simulink model "gm_receive_OK"  (R2015b)
settings: Solver=VariableStepAuto  StartTime=0  StopTime=25  RelTol=1e-3
settings Model: Creator=Administrator  LastModifiedBy=Administrator
settings OptimizationCC: BlockReduction=off  ConditionallyExecuteInputs=off
settings DebuggingCC: InheritedTsInSrcMsg=none

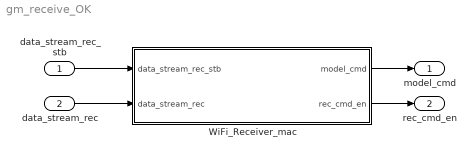
== system gm_receive_OK ==
  data_stream_rec_stb : Inport  OutDataTypeStr=boolean  SampleTime=0
  data_stream_rec : Inport  Port=2  OutDataTypeStr=uint8  SampleTime=0
  WiFi_Receiver_mac : Subsystem
  model_cmd : Outport  OutDataTypeStr=fixdt(0,4,0)
  rec_cmd_en : Outport  Port=2  OutDataTypeStr=boolean
  wires:
  data_stream_rec_stb/1 -> WiFi_Receiver_mac/1(data_stream_rec_stb)
  data_stream_rec/1 -> WiFi_Receiver_mac/2(data_stream_rec)
  WiFi_Receiver_mac/1(model_cmd) -> model_cmd/1
  WiFi_Receiver_mac/2(rec_cmd_en) -> rec_cmd_en/1

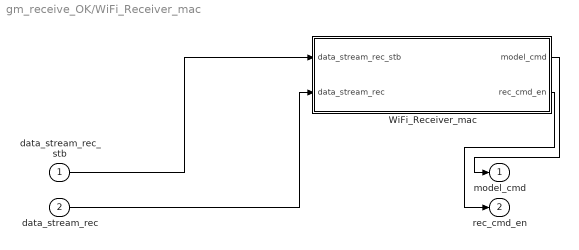
== system gm_receive_OK/WiFi_Receiver_mac ==
  data_stream_rec_stb : Inport  SampleTime=0
  data_stream_rec : Inport  Port=2  SampleTime=0
  WiFi_Receiver_mac : Stateflow chart  TreatAsAtomicUnit=on
  model_cmd : Outport
  rec_cmd_en : Outport  Port=2
  wires:
  data_stream_rec_stb/1 -> WiFi_Receiver_mac/1(data_stream_rec_stb)
  data_stream_rec/1 -> WiFi_Receiver_mac/2(data_stream_rec)
  WiFi_Receiver_mac/1(model_cmd) -> model_cmd/1
  WiFi_Receiver_mac/2(rec_cmd_en) -> rec_cmd_en/1

== stateflow chart gm_receive_OK/WiFi_Receiver_mac/WiFi_Receiver_mac ==
  settings: executeAtInitialization=1
  state wait_cmd
    entry:
    model_cmd=0;
    rec_cmd_en=0;
  state initial
    entry:
    model_cmd=0;
    rec_cmd_en=0;
    time_cnt=0;
  state received_OK
    entry:
    model_cmd=1;
    rec_cmd_en=1;
  state receive_Carriage_Return
  state detect_cmd
  state received_O
  state received_K
  state received_ERROR
    entry:
    model_cmd=2;
    rec_cmd_en=1;
  state time_out
    time_cnt=0;
    model_cmd=2;
    rec_cmd_en=1;
  state received_E
  state received_R
  state received_R1
  state received_O1
  state received_R2
  state receive_Carriage_Return1
  state received_FAIL
    entry:
    model_cmd=3;
    rec_cmd_en=1;
  state received_F
  state received_A
  state received_I
  state received_L
  state receive_Carriage_Return2
  (junction 129) -> wait_cmd
  (junction 152) -> (junction 129)
  (junction 13) -> (junction 129) [order 2] : [data_stream_rec~=75]
  (junction 150) -> (junction 152) [order 2] : [data_stream_rec~=13]
  (junction 22) -> wait_cmd : [(data_stream_rec~=79)&&(data_stream_rec~=69)&&(data_stream_rec~=70)]
  (junction 18) -> (junction 22) [order 2]
  (default) -> initial
  (junction 146) -> received_K [order 2] : [data_stream_rec_stb==0]
  (junction 10) -> received_O [order 1] : [data_stream_rec_stb==0]
  received_OK -> detect_cmd
  receive_Carriage_Return -> received_OK
  (junction 150) -> receive_Carriage_Return [order 1] : [data_stream_rec==13] %Carrage Return
  (junction 146) -> (junction 150) [order 1] : [data_stream_rec_stb==1]
  wait_cmd -> (junction 6)
  (junction 6) -> (junction 18) [order 1] : [data_stream_rec_stb==1]
  (junction 18) -> received_O [order 1] : [data_stream_rec==79]
  received_O -> (junction 10)
  (junction 10) -> (junction 13) [order 2] : [data_stream_rec_stb==1]
  (junction 13) -> received_K [order 1] : [data_stream_rec==75]
  received_K -> (junction 146)
  initial -> wait_cmd
  (junction 6) -> (junction 38) [order 2] : [data_stream_rec_stb==0]{time_cnt = time_cnt + 1;}
  (junction 18) -> (junction 52) [order 3]
  (junction 38) -> wait_cmd [order 2] : [time_cnt<=60000000]
  (junction 38) -> time_out [order 1] : [time_cnt>60000000]
  (junction 158) -> received_R2 [order 2] : [data_stream_rec_stb==0]
  (junction 79) -> received_O1 [order 2] : [data_stream_rec_stb==0]
  (junction 73) -> received_R1 [order 2] : [data_stream_rec_stb==0]
  (junction 66) -> received_R [order 2] : [data_stream_rec_stb==0]
  (junction 55) -> received_E [order 1] : [data_stream_rec_stb==0]
  receive_Carriage_Return1 -> received_ERROR
  received_ERROR -> detect_cmd
  received_E -> (junction 55)
  (junction 55) -> (junction 56) [order 2] : [data_stream_rec_stb==1]
  (junction 56) -> received_R [order 1] : [data_stream_rec==82]
  received_R -> (junction 66)
  (junction 66) -> (junction 64) [order 1] : [data_stream_rec_stb==1]
  (junction 64) -> received_R1 [order 1] : [data_stream_rec==82]
  received_R1 -> (junction 73)
  (junction 73) -> (junction 71) [order 1] : [data_stream_rec_stb==1]
  (junction 71) -> received_O1 [order 1] : [data_stream_rec==79]
  received_O1 -> (junction 79)
  (junction 79) -> (junction 77) [order 1] : [data_stream_rec_stb==1]
  (junction 77) -> received_R2 [order 1] : [data_stream_rec==82]
  (junction 165) -> receive_Carriage_Return1 [order 1] : [data_stream_rec==13] %Carrage Return
  (junction 52) -> received_E [order 1] : [data_stream_rec==69]
  (junction 158) -> (junction 165) [order 1] : [data_stream_rec_stb==1]
  received_R2 -> (junction 158)
  (junction 77) -> (junction 132) [order 2] : [data_stream_rec~=82]
  (junction 71) -> (junction 132) [order 2] : [data_stream_rec~=79]
  (junction 64) -> (junction 132) [order 2] : [data_stream_rec~=82]
  time_out -> wait_cmd
  (junction 52) -> (junction 124) [order 2]
  (junction 56) -> (junction 132) [order 2] : [data_stream_rec~=82]
  (junction 165) -> (junction 164) [order 2] : [data_stream_rec~=13]
  (junction 132) -> wait_cmd
  (junction 164) -> (junction 132)
  (junction 169) -> received_L [order 2] : [data_stream_rec_stb==0]
  (junction 97) -> received_I [order 2] : [data_stream_rec_stb==0]
  (junction 121) -> received_A [order 2] : [data_stream_rec_stb==0]
  (junction 123) -> received_F [order 1] : [data_stream_rec_stb==0]
  (junction 124) -> received_F : [data_stream_rec==70]
  received_F -> (junction 123)
  (junction 123) -> (junction 114) [order 2] : [data_stream_rec_stb==1]
  (junction 114) -> received_A [order 1] : [data_stream_rec==65]
  received_A -> (junction 121)
  (junction 121) -> (junction 119) [order 1] : [data_stream_rec_stb==1]
  (junction 119) -> received_I [order 1] : [data_stream_rec==73]
  received_I -> (junction 97)
  (junction 97) -> (junction 99) [order 1] : [data_stream_rec_stb==1]
  (junction 99) -> received_L [order 1] : [data_stream_rec==76]
  (junction 176) -> receive_Carriage_Return2 [order 1] : [data_stream_rec==13] %Carrage Return
  (junction 169) -> (junction 176) [order 1] : [data_stream_rec_stb==1]
  received_FAIL -> detect_cmd
  received_L -> (junction 169)
  (junction 99) -> (junction 138) [order 2] : [data_stream_rec~=76]
  (junction 119) -> (junction 138) [order 2] : [data_stream_rec~=73]
  receive_Carriage_Return2 -> received_FAIL
  (junction 114) -> (junction 138) [order 2] : [data_stream_rec~=65]
  (junction 176) -> (junction 175) [order 2] : [data_stream_rec~=13]
  (junction 175) -> (junction 138)
  (junction 138) -> wait_cmd
  detect_cmd -> (junction 32)
  (junction 34) -> wait_cmd
  (junction 32) -> (junction 34)
  data: data_stream_rec_stb input boolean; data_stream_rec input uint8; model_cmd output fixdt(0,4,0); rec_cmd_en output boolean; time_cnt local uint32
